simulink model "myrobot"  (R2019b)
settings: Solver=FixedStepAuto  StartTime=0.0  StopTime=2  FixedStep=0.001  MaxStep=0.005  RelTol=1e-3
values from neighbouring files (symbols this model uses):
  g = [0 0 -9.81]    [FK.m]    (also in FK_3DOF.m = [0 0 9.81])
  X = [joint1_pos(1) joint2_pos(1) joint3_pos(1) ee_pos(1)]    [plot_result.m]
  Y = [joint1_pos(2) joint2_pos(2) joint3_pos(2) ee_pos(2)]    [plot_result.m]
  Z = [joint1_pos(3) joint2_pos(3) joint3_pos(3) ee_pos(3)]    [plot_result.m]
libraries: sm_lib x17, nesl_utility x13, robotmaniplib x4, simulink x2
(part 7 of 7)

== matlab function myrobot/JOINT SPACE PASSIVITY BASED ADAPTIVE CONTROLLER/MATLAB Function5 ==
  data: t input; q input; q_dot input; a input; v input; r input; estimated_theta_dot output
function estimated_theta_dot = calc_estimated_theta_dot(t, q, q_dot, a, v, r)
    g = 9.81;
   
    Y = [ (q_dot(1)*v(2)*sin(2*q(2)))/2 - a(1)*(cos(2*q(2))/2 - 1/2) + (q_dot(2)*v(1)*sin(2*q(2)))/2, a(1)*sin(2*q(2)) + q_dot(1)*v(2)*cos(2*q(2)) + q_dot(2)*v(1)*cos(2*q(2)), v(1)*((q_dot(2)*sin(2*q(2) + 2*q(3)))/2 + (q_dot(3)*sin(2*q(2) + 2*q(3)))/2) - a(1)*(cos(2*q(2) + 2*q(3))/2 - 1/2) + (q_dot(1)*v(2)*sin(2*q(2) + 2*q(3)))/2 + (q_dot(1)*v(3)*sin(2*q(2) + 2*q(3)))/2, a(1)*(cos(2*q(2))/2 + 1/2) - (q_dot(1)*v(2)*sin(2*q(2)))/2 - (q_dot(2)*v(1)*sin(2*q(2)))/2, a(2)*sin(q(2)) + q_dot(2)*v(2)*cos(q(2)), a(1)*sin(2*q(2) + 2*q(3)) + v(1)*(q_dot(2)*cos(2*q(2) + 2*q(3)) + q_dot(3)*cos(2*q(2) + 2*q(3))) + q_dot(1)*v(2)*cos(2*q(2) + 2*q(3)) + q_dot(1)*v(3)*cos(2*q(2) + 2*q(3)), a(1), a(2)*cos(q(2)) - q_dot(2)*v(2)*sin(q(2)), a(1)*(cos(2*q(2) + 2*q(3))/2 + 1/2) - v(1)*((q_dot(2)*sin(2*q(2) + 2*q(3)))/2 + (q_dot(3)*sin(2*q(2) + 2*q(3)))/2) - (q_dot(1)*v(2)*sin(2*q(2) + 2*q(3)))/2 - (q_dot(1)*v(3)*sin(2*q(2) + 2*q(3)))/2, v(2)*(q_dot(2)*cos(q(2) + q(3)) + q_dot(3)*cos(q(2) + q(3))) + v(3)*(q_dot(2)*cos(q(2) + q(3)) + q_dot(3)*cos(q(2) + q(3))) + a(2)*sin(q(2) + q(3)) + a(3)*sin(q(2) + q(3)),  0, a(2)*cos(q(2) + q(3)) - v(3)*(q_dot(2)*sin(q(2) + q(3)) + q_dot(3)*sin(q(2) + q(3))) - v(2)*(q_dot(2)*sin(q(2) + q(3)) + q_dot(3)*sin(q(2) + q(3))) + a(3)*cos(q(2) + q(3)),       0,              0,              0,                       0, a(1), a(1), (q_dot(1)*v(2)*sin(2*q(2)))/2 - a(1)*(cos(2*q(2))/2 - 1/2) + (q_dot(2)*v(1)*sin(2*q(2)))/2, a(1), (q_dot(1)*v(2)*sin(2*q(2)))/2 - a(1)*(cos(2*q(2))/2 - 1/2) + (q_dot(2)*v(1)*sin(2*q(2)))/2, a(1), v(1)*((q_dot(2)*sin(2*q(2) + 2*q(3)))/2 + (q_dot(3)*sin(2*q(2) + 2*q(3)))/2) - a(1)*(cos(2*q(2) + 2*q(3))/2 - 1/2) + (q_dot(1)*v(2)*sin(2*q(2) + 2*q(3)))/2 + (q_dot(1)*v(3)*sin(2*q(2) + 2*q(3)))/2, a(1), q_dot(2)*v(2)*sin(q(2)) - a(2)*cos(q(2)), q_dot(2)*v(2)*sin(q(2)) - a(2)*cos(q(2)), 2*a(1), v(2)*(q_dot(2)*sin(q(2) + q(3)) + q_dot(3)*sin(q(2) + q(3))) + v(3)*(q_dot(2)*sin(q(2) + q(3)) + q_dot(3)*sin(q(2) + q(3))) - a(2)*cos(q(2) + q(3)) - a(3)*cos(q(2) + q(3)), 2*a(1), v(1)*(q_dot(2)*sin(2*q(2) + q(3)) + q_dot(3)*(sin(2*q(2) + q(3))/2 - sin(q(3))/2)) - a(1)*(cos(2*q(2) + q(3)) - cos(q(3))) - v(3)*((q_dot(1)*sin(q(3)))/2 - (q_dot(1)*sin(2*q(2) + q(3)))/2) + q_dot(1)*v(2)*sin(2*q(2) + q(3)), q_dot(2)*v(2)*sin(q(2)) - a(2)*cos(q(2)), q_dot(2)*v(2)*sin(q(2)) - a(2)*cos(q(2)), v(2)*(q_dot(2)*sin(q(2) + q(3)) + q_dot(3)*sin(q(2) + q(3))) + v(3)*(q_dot(2)*sin(q(2) + q(3)) + q_dot(3)*sin(q(2) + q(3))) - a(2)*cos(q(2) + q(3)) - a(3)*cos(q(2) + q(3));
                                                               -(q_dot(1)*v(1)*sin(2*q(2)))/2,                                                 -q_dot(1)*v(1)*cos(2*q(2)),                                                                                                                                                                              -(q_dot(1)*v(1)*sin(2*q(2) + 2*q(3)))/2,                                                                (q_dot(1)*v(1)*sin(2*q(2)))/2,                             a(1)*sin(q(2)),                                                                                                                                                        -q_dot(1)*v(1)*cos(2*q(2) + 2*q(3)),  0,                             a(1)*cos(q(2)),                                                                                                                                                                               (q_dot(1)*v(1)*sin(2*q(2) + 2*q(3)))/2,                                                                                                                                                                             a(1)*sin(q(2) + q(3)), a(2),                                                                                                                                                                             a(1)*cos(q(2) + q(3)), a(2) + a(3), -g*sin(q(2)), -g*sin(q(2)), -g*sin(q(2) + q(3)),  0,  0,                                                           a(2) - (q_dot(1)*v(1)*sin(2*q(2)))/2,  0,                                                           a(2) - (q_dot(1)*v(1)*sin(2*q(2)))/2,  0,                                                                                                                                                                     a(2) + a(3) - (q_dot(1)*v(1)*sin(2*q(2) + 2*q(3)))/2,  0,                            -a(1)*cos(q(2)),                            -a(1)*cos(q(2)),    0,                                                                                                                                                                            -a(1)*cos(q(2) + q(3)),    0,                                                                                                             2*a(2)*cos(q(3)) + a(3)*cos(q(3)) - v(3)*sin(q(3))*(q_dot(2) + q_dot(3)) - q_dot(3)*v(2)*sin(q(3)) - q_dot(1)*v(1)*sin(2*q(2) + q(3)),                            -a(1)*cos(q(2)),                            -a(1)*cos(q(2)),                                                                                                                                                                            -a(1)*cos(q(2) + q(3));
                                                                                              0,                                                                            0,                                                                                                                                                                              -(q_dot(1)*v(1)*sin(2*q(2) + 2*q(3)))/2,                                                                                              0,                                          0,                                                                                                                                                        -q_dot(1)*v(1)*cos(2*q(2) + 2*q(3)),  0,                                          0,                                                                                                                                                                               (q_dot(1)*v(1)*sin(2*q(2) + 2*q(3)))/2,                                                                                                                                                                             a(1)*sin(q(2) + q(3)),  0,                                                                                                                                                                             a(1)*cos(q(2) + q(3)), a(2) + a(3),              0,              0, -g*sin(q(2) + q(3)),  0,  0,                                                                                              0,  0,                                                                                              0,  0,                                                                                                                                                                     a(2) + a(3) - (q_dot(1)*v(1)*sin(2*q(2) + 2*q(3)))/2,  0,                                          0,                                          0,    0,                                                                                                                                                                            -a(1)*cos(q(2) + q(3)),    0,                                                                                                                                                       a(2)*cos(q(3)) + q_dot(2)*v(2)*sin(q(3)) - q_dot(1)*v(1)*(sin(2*q(2) + q(3))/2 - sin(q(3))/2),                                          0,                                          0,                                                                                                                                                                            -a(1)*cos(q(2) + q(3))];
    %----- PARAMETER TO TUNE -----%
    gamma = 200; % SMALL GAIN - FAST RESPONSE
    %-----------------------------%
    if (t > 0.002)
        estimated_theta_dot = -inv(gamma) * Y' * r;
    else 
        estimated_theta_dot = zeros(33,1);
    end
end
